simulink model "inner_PD_angle_d"  (R2018a)
settings: Solver=FixedStepAuto  StartTime=0.0  StopTime=10  RelTol=1e-3  EnableMultiTasking=on

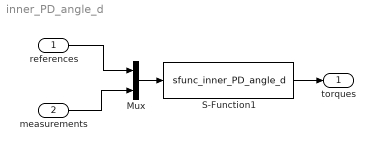
== system inner_PD_angle_d ==
  references : Inport  PortDimensions=12
  measurements : Inport  Port=2  PortDimensions=12
  Mux : Mux  Inputs=2
  S-Function1 : S-Function  FunctionName=sfunc_inner_PD_angle_d  Parameters=PD_angle_param  SFunctionDeploymentMode=off  EnableBusSupport=off
  torques : Outport
  wires:
  measurements/1 -> Mux/2
  references/1 -> Mux/1
  Mux/1 -> S-Function1/1
  S-Function1/1 -> torques/1
